simulink model "Simulink_Model_adaptive_Impedance"  (R2023b)
settings: Solver=VariableStepAuto  StartTime=0.0  StopTime=10.0  RelTol=1e-3
settings Model: Creator=91996  LastModifiedBy=Dell

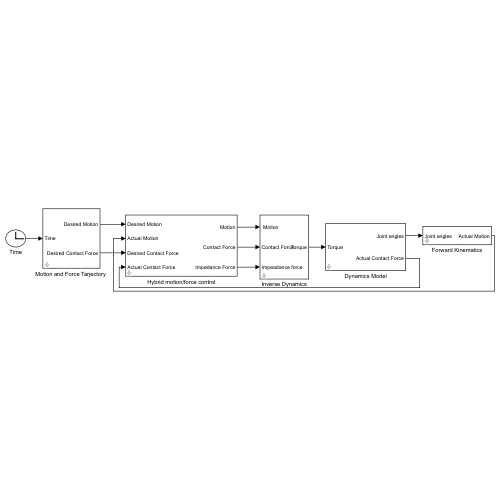
[thumbnail: Simulink's stored preview of the top-level diagram]
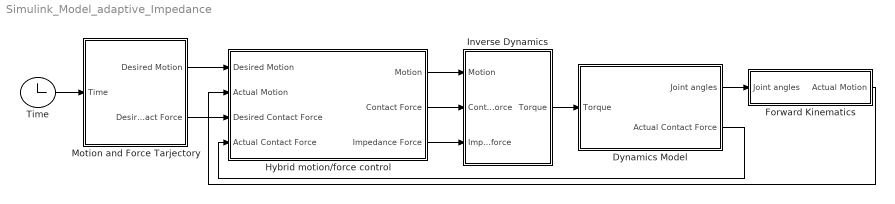
== system Simulink_Model_adaptive_Impedance ==
  Dynamics Model : Subsystem
      mask DialogControl C Prompt: Parameters
  Forward Kinematics : Subsystem
      mask DialogControl Kinematics Prompt: Parameters
  Hybrid motion/force control : Subsystem
      mask DialogControl A Prompt: Parameters
  Inverse Dynamics : Subsystem
      mask DialogControl B Prompt: Parameters
  "Motion and Force Tarjectory " : Subsystem
      mask DialogControl E Prompt: Parameters
  Time : Clock
  wires:
  "Motion and Force Tarjectory "/1(Desired Motion) -> Hybrid motion/force control/1(Desired Motion)
  Hybrid motion/force control/1(" Motion") -> Inverse Dynamics/1(" Motion")
  Time/1 -> "Motion and Force Tarjectory "/1(Time)
  Inverse Dynamics/1(Torque) -> Dynamics Model/1(Torque)
  Forward Kinematics/1(Actual Motion) -> Hybrid motion/force control/2(Actual Motion)
  Dynamics Model/1(Joint angles) -> Forward Kinematics/1(Joint angles)
  "Motion and Force Tarjectory "/2(Desired Contact Force) -> Hybrid motion/force control/3(Desired Contact Force)
  Dynamics Model/2(Actual Contact Force) -> Hybrid motion/force control/4(Actual Contact Force)
  Hybrid motion/force control/2(Contact Force) -> Inverse Dynamics/2(Contact Force)
  Hybrid motion/force control/3(Impedance Force) -> Inverse Dynamics/3(Impeadance force)

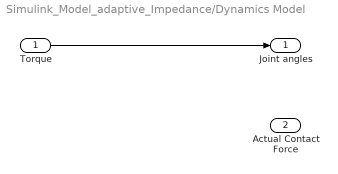
== system Simulink_Model_adaptive_Impedance/Dynamics Model ==
  Torque : Inport
  Joint angles : Outport
  Actual Contact Force : Outport  Port=2
  wires:
  Torque/1 -> Joint angles/1

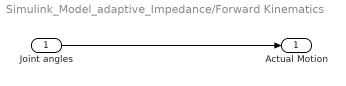
== system Simulink_Model_adaptive_Impedance/Forward Kinematics ==
  Joint angles : Inport
  Actual Motion : Outport
  wires:
  Joint angles/1 -> Actual Motion/1

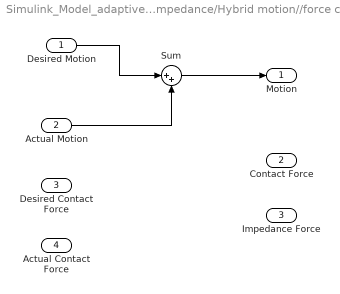
== system Simulink_Model_adaptive_Impedance/Hybrid motion//force control ==
  Desired Motion : Inport
  Actual Motion : Inport  Port=2
  Desired Contact Force : Inport  Port=3
  Actual Contact Force : Inport  Port=4
  Sum : Sum  Inputs=|++
  " Motion" : Outport
  Contact Force : Outport  Port=2
  Impedance Force : Outport  Port=3
  wires:
  Desired Motion/1 -> Sum/1
  Actual Motion/1 -> Sum/2
  Sum/1 -> " Motion"/1

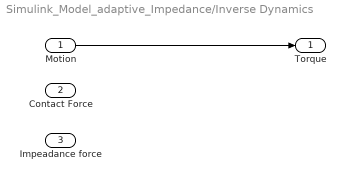
== system Simulink_Model_adaptive_Impedance/Inverse Dynamics ==
  " Motion" : Inport
  Contact Force : Inport  Port=2
  Impeadance force : Inport  Port=3
  Torque : Outport
  wires:
  " Motion"/1 -> Torque/1

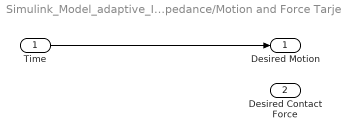
== system Simulink_Model_adaptive_Impedance/Motion and Force Tarjectory  ==
  Time : Inport
  Desired Motion : Outport
  Desired Contact Force : Outport  Port=2
  wires:
  Time/1 -> Desired Motion/1
